simulink model "Multiuav"  (Simulink 4.00)
settings: Solver=FixedStepDiscrete  StartTime=0.0  StopTime=g_StopTime  FixedStep=g_SampleTime  RelTol=1e-3
undefined symbols (not defined in the file): ATRFunctions, g_AssignmentAlgorithm, g_CommandTurnRadius, g_CoordinationDelayDen, g_DefaultWaypointAltitude, g_EnableTarget, g_EnableVehicle, g_EntityTypes, g_MaxNumberTargets, g_MaxNumberVehicles, g_MaxReassignmentDeltaTime, g_ObjectMessageIDs, g_OptionSaveDataAVDS, g_OptionSaveDataPlot, g_SampleTime, g_SensorRollLimitDeg, g_TargetStates, g_Tasks, g_TypeAssignment, g_VehicleInputFiles, g_VehicleMemory, g_VehicleTypes, g_WaypointDefinitions, g_WaypointTypes
libraries: cooperative x42
(part 2 of 4)

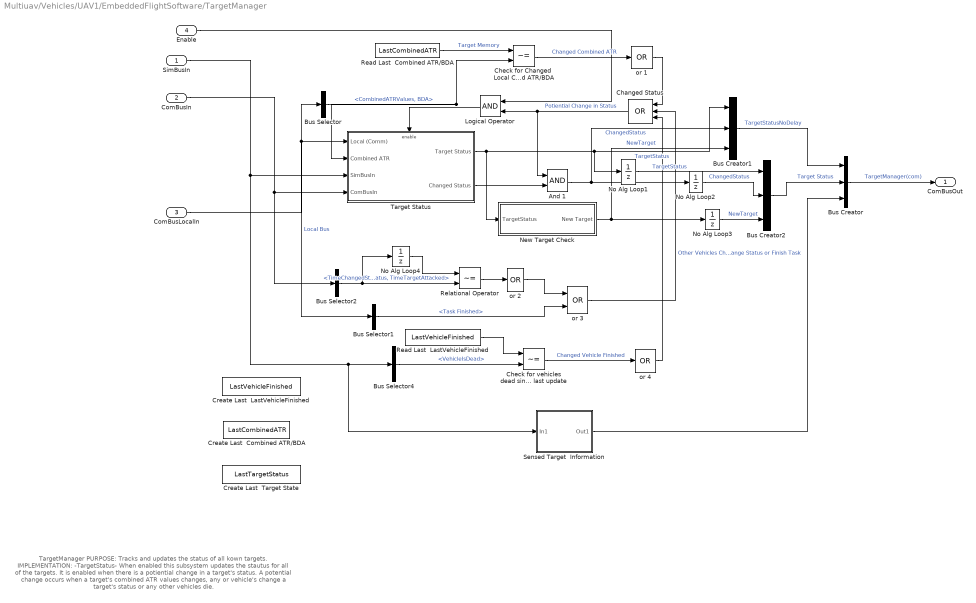
== system Multiuav/Vehicles/UAV1/EmbeddedFlightSoftware/TargetManager ==
  note: TargetManager
      |
      | PURPOSE: Tracks and updates the status of all
      |      kown targets.
      |
      | IMPLEMENTATION:
      | -TargetStatus- When enabled this subsystem updates the stautus for all of the targets.
      |      It is enabled when there is a potiential change in a target's status. A potential
      |      change occurs when a target's combined ATR values changes, any or vehicle's
      |      change a target's status or any other vehicles die.
  SimBusIn : Inport  Port=1  LatchInput=off  SampleTime=g_SampleTime
  ComBusIn : Inport  Port=2  LatchInput=off  SampleTime=g_SampleTime
  ComBusLocalIn : Inport  Port=3  LatchInput=off  SampleTime=g_SampleTime
  Enable : Inport  Port=4  LatchInput=off  SampleTime=g_SampleTime
  And 1 : Logic  Operator=AND  Inputs=2
  Bus Creator : BusCreator  Inputs=3
  Bus Creator1 : BusCreator  Inputs=3
  Bus Creator2 : BusCreator  Inputs=3
  Bus Selector : BusSelector  OutputSignals=EFS(com).SensorManager(com).ATR Combined.CombinedATRValues,EFS(com).SensorManager(com).BDA  MuxedOutput=on
  Bus Selector1 : BusSelector  OutputSignals=EFS(com).RouteManager(com).TaskStatus.Task Finished  MuxedOutput=off
  Bus Selector2 : BusSelector  OutputSignals=TimeChangedStatus,TimeTargetAttacked  MuxedOutput=on
  Bus Selector4 : BusSelector  OutputSignals=ExternalTruth.VehicleIsDead  MuxedOutput=on
  Changed Status : Logic  Orientation=left  Operator=OR  Inputs=3
  Check for Changed  Local Combined ATR/BDA : RelationalOperator  Operator=~=
  Check for vehicles dead since last update : RelationalOperator  Operator=~=
  Create Last  Combined ATR/BDA : DataStoreMemory  DataStoreName=LastCombinedATR  InitialValue=[1:(g_MaxNumberTargets*2)]*0
  Create Last  LastVehicleFinished : DataStoreMemory  DataStoreName=LastVehicleFinished  InitialValue=[1:(g_MaxNumberVehicles)]*0
  Create Last  Target State : DataStoreMemory  DataStoreName=LastTargetStatus  InitialValue=[1:(g_MaxNumberTargets)]*0
  Logical Operator : Logic  Orientation=left  Operator=AND  Inputs=2
  New Target Check : Subsystem
      settings: RTWFcnNameOpts=Auto  RTWFileNameOpts=Auto
  No Alg Loop{1..4} (4 alike) : UnitDelay  X0=0  SampleTime=g_SampleTime
      settings: RTWStateStorageClass=Auto
  Read Last  Combined ATR/BDA : DataStoreRead  DataStoreName=LastCombinedATR  SampleTime=g_SampleTime
  Read Last  LastVehicleFinished : DataStoreRead  DataStoreName=LastVehicleFinished  SampleTime=g_SampleTime
  Relational Operator : RelationalOperator  Operator=~=
  Sensed Target  Information : Subsystem
      settings: RTWFcnNameOpts=Auto  RTWFileNameOpts=Auto
  Target Status : Subsystem  TreatAsAtomicUnit=on
      settings: RTWFcnNameOpts=Auto  RTWFileNameOpts=Auto
  or 1 : Logic  Operator=OR  Inputs=1
  or 2 : Logic  Operator=OR  Inputs=1
  or 3 : Logic  Operator=OR  Inputs=2
  or 4 : Logic  Operator=OR  Inputs=1
  ComBusOut : Outport  Port=1
  wires:
  or 2/1 -> or 3/1
  No Alg Loop4/1 -> Relational Operator/1
  No Alg Loop3/1 -> Bus Creator2/3  "NewTarget"
  No Alg Loop2/1 -> Bus Creator2/2  "ChangedStatus"
  No Alg Loop1/1 -> Bus Creator2/1  "TargetStatus"
  New Target Check/1(New Target) -> No Alg Loop3/1, Bus Creator1/3  "NewTarget"
  Sensed Target  Information/1(Out1) -> Bus Creator/3
  Enable/1 -> Logical Operator/1
  Logical Operator/1 -> Target Status/Enable
  Bus Selector4/1 -> Check for vehicles dead since last update/2  "<VehicleIsDead>"
  Read Last  LastVehicleFinished/1 -> Check for vehicles dead since last update/1
  Check for vehicles dead since last update/1 -> or 4/1  "Changed Vehicle Finished"
  or 4/1 -> Changed Status/3
  or 3/1 -> Changed Status/2  "Other Vehicles Change Status or Finish Task"
  Relational Operator/1 -> or 2/1
  Bus Selector1/1 -> or 3/2  "<Task Finished>"
  Check for Changed  Local Combined ATR/BDA/1 -> or 1/1  "Changed Combined ATR"
  Target Status/1(Target Status) -> No Alg Loop1/1, Bus Creator1/1, New Target Check/1(TargetStatus)  "TargetStatus"
  Bus Creator2/1 -> Bus Creator/2  "Target Status"
  Changed Status/1 -> Logical Operator/2, And 1/1  "Potiential Change in Status"
  Bus Selector2/1 -> Relational Operator/2, No Alg Loop4/1  "<TimeChangedStatus, TimeTargetAttacked>"
  or 1/1 -> Changed Status/1
  Bus Selector/1 -> Target Status/2(Combined ATR), Check for Changed  Local Combined ATR/BDA/2  "<CombinedATRValues, BDA>"
  Read Last  Combined ATR/BDA/1 -> Check for Changed  Local Combined ATR/BDA/1  "Target Memory"
  Target Status/2(Changed Status) -> And 1/2
  And 1/1 -> Bus Creator1/2, No Alg Loop2/1  "ChangedStatus"
  ComBusIn/1 -> Bus Selector2/1, Target Status/4(ComBusIn)
  Bus Creator/1 -> ComBusOut/1  "TargetManager(com)"
  SimBusIn/1 -> Sensed Target  Information/1(In1), Bus Selector4/1, Target Status/3(SimBusIn)
  ComBusLocalIn/1 -> Bus Selector1/1, Bus Selector/1, Target Status/1(Local (Comm))  "Local Bus"
  Bus Creator1/1 -> Bus Creator/1  "TargetStatusNoDelay"

== system Multiuav/Vehicles/UAV1/EmbeddedFlightSoftware/WeaponsManager ==
  note: Weapons Manager
      |
      | PURPOSE: Selects a weapon and then simulates its deployment.
      |
      | IMPLEMENTATION:
      | -TargetBombed- calls the function "WeaponsRelease.m" which returns
      |      a unique BombID number, the type of bomb dropped and the
      |      bomb's impact coordinates.
  ComBusLocalIn : Inport  Port=1  LatchInput=off  SampleTime=g_SampleTime
  Enable : EnablePort
  Bus Creator : BusCreator  Inputs=1
  Bus Creator1 : BusCreator  Inputs=1
  Bus Creator2 : BusCreator  Inputs=4
  Bus Selector : BusSelector  OutputSignals=VehicleID,EFS(com).RouteManager(com).TaskStatus.Target Attacked,Dynamics(com).AC Dynamics.Position_x,Dynamics(com).AC Dynamics.Position_y  MuxedOutput=on
  Constant : Constant  Value=0
  Demux : Demux  Outputs=4  BusSelectionMode=off
  TargetBombed : S-Function  FunctionName=WeaponsReleaseS  Parameters='Bomb'  PortCounts=[]  SFunctionModules=''
  SimBusOut : Outport  Port=1
  ComBusOut : Outport  Port=2  InitialOutput=[0]
  wires:
  Bus Selector/1 -> TargetBombed/1  "<VehicleID, Target Attacked, Position_x, Position_y>"
  Bus Creator2/1 -> Bus Creator1/1  "BombDrop"
  Bus Creator1/1 -> SimBusOut/1  "WeaponsManager(sim)"
  Demux/4 -> Bus Creator2/4  "BombPositionY"
  Demux/3 -> Bus Creator2/3  "BombPositionX"
  Demux/2 -> Bus Creator2/2  "BombType"
  Demux/1 -> Bus Creator2/1  "BombID"
  TargetBombed/1 -> Demux/1
  Constant/1 -> Bus Creator/1  "WeaponsManagerTemp"
  Bus Creator/1 -> ComBusOut/1  "WeaponsManager(com)"
  ComBusLocalIn/1 -> Bus Selector/1

== system Multiuav/Vehicles/UAV1/ReceiveTruth/ImplementNewAssignment ==
  VehicleID : Inport  Port=1  LatchInput=off
  TruthBus : Inport  Port=2  LatchInput=off
  Constant : Constant  Value=0
  Relational Operator : RelationalOperator  Operator=<
  VehicleAlive : Subsystem  TreatAsAtomicUnit=on
      settings: RTWFcnNameOpts=Auto  RTWFileNameOpts=Auto
  wires:
  TruthBus/1 -> VehicleAlive/2(In2)
  Constant/1 -> Relational Operator/1
  VehicleID/1 -> VehicleAlive/1(In1), Relational Operator/2
  Relational Operator/1 -> VehicleAlive/Enable

== system Multiuav/Vehicles/UAV1/SaveAVDSData/SaveVehicleData for AVDS ==
  note: SaveVehicleData for AVDS
      |
      | PURPOSE: Saves vehicle state information to a text file that is suitable
      |      for playback in AVDS.
      | IMPLEMENTATION:
      | - AVDSData2WorkSpace - calls the M-function "AVDSData2WorkSpace"
      |      to save the data.
  Time : Inport  Port=1  LatchInput=off  SampleTime=g_SampleTime
  ID : Inport  Port=2  LatchInput=off  SampleTime=g_SampleTime
  Data : Inport  Port=3  LatchInput=off  SampleTime=g_SampleTime
  Vehicle Type : Inport  Port=4  LatchInput=off  SampleTime=g_SampleTime
  Enable : EnablePort
  AVDSData2WorkSpaceS : S-Function  FunctionName=AVDSData2WorkSpaceS  PortCounts=[]  SFunctionModules=''
  Mux1 : Mux  Inputs=4
  wires:
  Vehicle Type/1 -> Mux1/4
  Data/1 -> Mux1/3
  ID/1 -> Mux1/1
  Time/1 -> Mux1/2
  Mux1/1 -> AVDSData2WorkSpaceS/1

== system Multiuav/Vehicles/UAV1/SendMessages/SendATRSingle ==
  VehicleID : Inport  Port=1  LatchInput=off
  CommBusLocal : Inport  Port=2  LatchInput=off
  Bus Selector4 : BusSelector  OutputSignals=EFS(com).SensorManager(com).ATR Single.ATR Time,EFS(com).SensorManager(com).ATR Single  MuxedOutput=on
  Mux3 : Mux  Inputs=3
  SendATRSingle : cooperative/SendMessage  ReuseMatrix=growing  MessageTypeStr=ATRSingle
  Terminator : Terminator
  VehicleOffset : Constant  Value=g_ObjectMessageIDs.AllVehiclesTypeShifted + 1
  wires:
  CommBusLocal/1 -> Bus Selector4/1
  VehicleID/1 -> Mux3/1
  Mux3/1 -> SendATRSingle/1
  Bus Selector4/1 -> Mux3/2  "<ATR Time, ATR Single>"
  VehicleOffset/1 -> Mux3/3
  SendATRSingle/1 -> Terminator/1

== system Multiuav/Vehicles/UAV1/SendMessages/SendATRTime ==
  VehicleID : Inport  Port=1  LatchInput=off
  CommBusLocal : Inport  Port=2  LatchInput=off
  Bus Selector1 : BusSelector  OutputSignals=EFS(com).SensorManager(com).ATR Single.ATR Time  MuxedOutput=off
  CreateWaypointIndex : DataStoreMemory  DataStoreName=ATRTime  InitialValue=0
  Enabled Subsystem : Subsystem  TreatAsAtomicUnit=on
      settings: RTWFcnNameOpts=Auto  RTWFileNameOpts=Auto
  Mux2 : Mux  Inputs=4
  ReadWaypointIndex : DataStoreRead  DataStoreName=ATRTime  SampleTime=g_SampleTime
  Relational Operator : RelationalOperator  Operator=~=
  SendATRTime : cooperative/SendMessage  ReuseMatrix=growing  MessageTypeStr=ATRTime
  Terminator : Terminator
  VehicleOffset : Constant  Value=g_ObjectMessageIDs.AllVehiclesTypeShifted + 1
  wires:
  Bus Selector1/1 -> Enabled Subsystem/1(ATRTime), Relational Operator/2, Mux2/3  "<ATR Time>"
  Enabled Subsystem/1(TimeStamp) -> Mux2/2  "TimeStamp"
  Mux2/1 -> SendATRTime/1
  Relational Operator/1 -> Enabled Subsystem/Enable
  ReadWaypointIndex/1 -> Relational Operator/1
  VehicleID/1 -> Mux2/1
  CommBusLocal/1 -> Bus Selector1/1
  VehicleOffset/1 -> Mux2/4
  SendATRTime/1 -> Terminator/1

== system Multiuav/Vehicles/UAV1/SendMessages/SendAuctionData ==
  VehicleID : Inport  Port=1  LatchInput=off
  CommBusLocal : Inport  Port=2  LatchInput=off
  Bus Selector1 : BusSelector  OutputSignals=EFS(com).CooperationManager(com).AuctionData.MessageNumber,EFS(com).CooperationManager(com).AuctionData.ReplanRound,EFS(com).CooperationManager(com).AuctionData.BidTarget,EFS(com).CooperationManager(com).AuctionData.BidPrice,EFS(com).CooperationManager(com).AuctionData.BidTargetETA,EFS(com).CooperationManager(com).AuctionData.AssignedTarget,EFS(com).CooperationManager(com).AuctionData.AssignedPrice,EFS(com).CooperationManager(com).AuctionData.AssignedTargetETA  MuxedOutput=off
  Data Store Memory : DataStoreMemory  DataStoreName=LastMessageNumber  InitialValue=0
  Data Store Read : DataStoreRead  DataStoreName=LastMessageNumber  SampleTime=g_SampleTime
  Enabled Subsystem : Subsystem  Priority=1  TreatAsAtomicUnit=on
      settings: RTWFcnNameOpts=Auto  RTWFileNameOpts=Auto
  Mux2 : Mux  Inputs=11
  Relational Operator : RelationalOperator  Operator=~=
  "SendAuctionData " : cooperative/SendMessage  Priority=2  ReuseMatrix=growing  MessageTypeStr=AuctionData
  Sum : Sum  Inputs=+  SaturateOnIntegerOverflow=on
  Terminator : Terminator
  VehicleOffset : Constant  Value=g_ObjectMessageIDs.AllVehiclesTypeShifted + 1
  wires:
  Bus Selector1/1 -> Enabled Subsystem/1(MessageNumber), Relational Operator/2  "<MessageNumber>"
  Bus Selector1/2 -> Mux2/4  "<ReplanRound>"
  Bus Selector1/3 -> Mux2/5  "<BidTarget>"
  Bus Selector1/4 -> Mux2/6  "<BidPrice>"
  Bus Selector1/5 -> Mux2/7  "<BidTargetETA>"
  Bus Selector1/6 -> Mux2/8  "<AssignedTarget>"
  Bus Selector1/7 -> Mux2/9  "<AssignedPrice>"
  Bus Selector1/8 -> Mux2/10  "<AssignedTargetETA>"
  Sum/1 -> Enabled Subsystem/Enable
  Relational Operator/1 -> Sum/1
  Data Store Read/1 -> Relational Operator/1
  Enabled Subsystem/1(TimeStamp) -> Mux2/3, Mux2/2  "TimeStamp"
  Mux2/1 -> "SendAuctionData "/1
  VehicleID/1 -> Mux2/1
  CommBusLocal/1 -> Bus Selector1/1
  VehicleOffset/1 -> Mux2/11
  "SendAuctionData "/1 -> Terminator/1

== system Multiuav/Vehicles/UAV1/SendMessages/SendChangedStatus ==
  VehicleID : Inport  Port=1  LatchInput=off
  CommBusLocal : Inport  Port=2  LatchInput=off
  Bus Selector1 : BusSelector  OutputSignals=EFS(com).TargetManager(com).Target Status.ChangedStatus  MuxedOutput=off
  Enabled Subsystem : Subsystem  TreatAsAtomicUnit=on
      settings: RTWFcnNameOpts=Auto  RTWFileNameOpts=Auto
  Mux2 : Mux  Inputs=4
  "SendChangedStatus " : cooperative/SendMessage  ReuseMatrix=growing  MessageTypeStr=ChangedStatus
  Terminator : Terminator
  VehicleOffset : Constant  Value=g_ObjectMessageIDs.AllVehiclesTypeShifted + 1
  wires:
  Bus Selector1/1 -> Enabled Subsystem/Enable, Mux2/3  "<ChangedStatus>"
  Enabled Subsystem/1(TimeStamp) -> Mux2/2  "TimeStamp"
  Mux2/1 -> "SendChangedStatus "/1
  VehicleID/1 -> Mux2/1
  CommBusLocal/1 -> Bus Selector1/1
  VehicleOffset/1 -> Mux2/4
  "SendChangedStatus "/1 -> Terminator/1

== system Multiuav/Vehicles/UAV1/SendMessages/SendETAsCostsReturnToSearch ==
  VehicleID : Inport  Port=1  LatchInput=off
  CommBusLocal : Inport  Port=2  LatchInput=off
  Bus Selector2 : BusSelector  OutputSignals=EFS(com).RouteManager(com).Replan ETAs and Costs.ReplanTime,EFS(com).RouteManager(com).Replan ETAs and Costs  MuxedOutput=on
  Mux : Mux  Inputs=3
  SendETAsCostsReturnToSearch : cooperative/SendMessage  ReuseMatrix=growing  MessageTypeStr=ETACostToSearch
  Terminator : Terminator
  VehicleOffset : Constant  Value=g_ObjectMessageIDs.AllVehiclesTypeShifted + 1
  wires:
  CommBusLocal/1 -> Bus Selector2/1
  VehicleID/1 -> Mux/1
  Mux/1 -> SendETAsCostsReturnToSearch/1
  Bus Selector2/1 -> Mux/2  "<ReplanTime, Replan ETAs and Costs>"
  VehicleOffset/1 -> Mux/3
  SendETAsCostsReturnToSearch/1 -> Terminator/1

== system Multiuav/Vehicles/UAV1/SendMessages/SendPositionFlag ==
  VehicleID : Inport  Port=1  LatchInput=off
  CommBusLocal : Inport  Port=2  LatchInput=off
  CommBus : Inport  Port=3  LatchInput=off
  Bus Selector1 : BusSelector  OutputSignals=EFS(com).TargetManager(com).Target Status.NewTarget,EFS(com).RouteManager(com).NewPlans  MuxedOutput=on
  Bus Selector2 : BusSelector  OutputSignals=TimeTriggerReplan  MuxedOutput=on
  CreateWaypointIndex : DataStoreMemory  DataStoreName=PositionFlag  InitialValue=[0 0 0]
  Enabled Subsystem : Subsystem  TreatAsAtomicUnit=on
      settings: RTWFcnNameOpts=Auto  RTWFileNameOpts=Auto
  Logical Operator1 : Logic  Operator=OR  Inputs=1
  Mux : Mux  Inputs=2
  Mux2 : Mux  Inputs=4
  ReadWaypointIndex : DataStoreRead  DataStoreName=PositionFlag  SampleTime=g_SampleTime
  Relational Operator : RelationalOperator  Operator=~=
  SendATRTime : cooperative/SendMessage  ReuseMatrix=growing  MessageTypeStr=SendPositionsFlag
  Terminator : Terminator
  VehicleOffset : Constant  Value=g_ObjectMessageIDs.AllVehiclesTypeShifted + 1
  wires:
  Mux/1 -> Enabled Subsystem/1(PositionFlag), Relational Operator/2
  Bus Selector1/1 -> Mux/1  "<NewTarget, NewPlans>"
  Bus Selector2/1 -> Mux/2  "<TimeTriggerReplan>"
  CommBus/1 -> Bus Selector2/1
  Logical Operator1/1 -> Mux2/3, Enabled Subsystem/Enable
  Relational Operator/1 -> Logical Operator1/1
  CommBusLocal/1 -> Bus Selector1/1
  VehicleID/1 -> Mux2/1
  ReadWaypointIndex/1 -> Relational Operator/1
  Mux2/1 -> SendATRTime/1
  Enabled Subsystem/1(TimeStamp) -> Mux2/2  "TimeStamp"
  VehicleOffset/1 -> Mux2/4
  SendATRTime/1 -> Terminator/1

== system Multiuav/Vehicles/UAV1/SendMessages/SendPositionID ==
  note: NOTE: Since the received messages are not reset to zero after they are handled, it was necessary to reset the PositionsFlag signal here.
      | The issue of resetting the message values to zero may be moved into the S-Function.
  VehicleID : Inport  Port=1  LatchInput=off
  CommBusLocal : Inport  Port=2  LatchInput=off
  CommBus : Inport  Port=3  LatchInput=off
  Bus Selector1 : BusSelector  OutputSignals=Dynamics(com).AC Dynamics.Position_x,Dynamics(com).AC Dynamics.Position_y,Dynamics(com).AC Dynamics.Psi  MuxedOutput=on
  Bus Selector2 : BusSelector  OutputSignals=TimePositionsFlag  MuxedOutput=on
  Data Store Memory : DataStoreMemory  DataStoreName=PositionsSendFlagTime  InitialValue=0
  Data Store Read : DataStoreRead  DataStoreName=PositionsSendFlagTime  SampleTime=g_SampleTime
  Enabled Subsystem : Subsystem  TreatAsAtomicUnit=on
      settings: RTWFcnNameOpts=Auto  RTWFileNameOpts=Auto
  Mux2 : Mux  Inputs=5
  Relational Operator : RelationalOperator  Operator=~=
  "SendPositionID " : cooperative/SendMessage  ReuseMatrix=growing  MessageTypeStr=PositionID
  Terminator : Terminator
  VehicleOffset : Constant  Value=g_ObjectMessageIDs.AllVehiclesTypeShifted + 1
  wires:
  Relational Operator/1 -> Enabled Subsystem/Enable
  Data Store Read/1 -> Relational Operator/1
  Bus Selector2/1 -> Relational Operator/2, Enabled Subsystem/1(PositionSendFlag Time)  "<TimePositionsFlag>"
  CommBus/1 -> Bus Selector2/1
  CommBusLocal/1 -> Bus Selector1/1
  VehicleID/1 -> Mux2/3, Mux2/1
  Mux2/1 -> "SendPositionID "/1
  Enabled Subsystem/1(TimeStamp) -> Mux2/2  "TimeStamp"
  Bus Selector1/1 -> Mux2/4  "<Position_x, Position_y, Psi>"
  VehicleOffset/1 -> Mux2/5
  "SendPositionID "/1 -> Terminator/1

== system Multiuav/Vehicles/UAV1/SendMessages/SendTargetAttacked ==
  VehicleID : Inport  Port=1  LatchInput=off
  CommBusLocal : Inport  Port=2  LatchInput=off
  Bus Selector1 : BusSelector  OutputSignals=EFS(com).RouteManager(com).TaskStatus.Target Attacked  MuxedOutput=off
  CreateWaypointIndex : DataStoreMemory  DataStoreName=TargetAttacked  InitialValue=0
  Enabled Subsystem : Subsystem  TreatAsAtomicUnit=on
      settings: RTWFcnNameOpts=Auto  RTWFileNameOpts=Auto
  Mux2 : Mux  Inputs=4
  ReadWaypointIndex : DataStoreRead  DataStoreName=TargetAttacked  SampleTime=g_SampleTime
  Relational Operator : RelationalOperator  Operator=~=
  "SendTargetAttacked " : cooperative/SendMessage  ReuseMatrix=growing  MessageTypeStr=TargetAttacked
  Terminator : Terminator
  VehicleOffset : Constant  Value=g_ObjectMessageIDs.AllVehiclesTypeShifted + 1
  wires:
  CommBusLocal/1 -> Bus Selector1/1
  VehicleID/1 -> Mux2/1
  ReadWaypointIndex/1 -> Relational Operator/1
  Relational Operator/1 -> Enabled Subsystem/Enable
  Mux2/1 -> "SendTargetAttacked "/1
  Enabled Subsystem/1(TimeStamp) -> Mux2/2  "TimeStamp"
  Bus Selector1/1 -> Mux2/3, Relational Operator/2, Enabled Subsystem/1("TargetAttacked ")  "<Target Attacked>"
  VehicleOffset/1 -> Mux2/4
  "SendTargetAttacked "/1 -> Terminator/1

== system Multiuav/Vehicles/UAV1/SendMessages/SendTargetStatus ==
  VehicleID : Inport  Port=1  LatchInput=off
  CommBusLocal : Inport  Port=2  LatchInput=off
  Bus Selector1 : BusSelector  OutputSignals=EFS(com).TargetManager(com).TargetStatusNoDelay.TargetStatus  MuxedOutput=off
  Bus Selector2 : BusSelector  OutputSignals=EFS(com).TargetManager(com).TargetStatusNoDelay.ChangedStatus  MuxedOutput=off
  Enabled Subsystem : Subsystem  Priority=1  TreatAsAtomicUnit=on
      settings: RTWFcnNameOpts=Auto  RTWFileNameOpts=Auto
  Mux2 : Mux  Inputs=4
  "SendTargetStatus " : cooperative/SendMessage  Priority=2  ReuseMatrix=growing  MessageTypeStr=TargetStatus
  Terminator : Terminator
  VehicleOffset : Constant  Value=g_ObjectMessageIDs.AllVehiclesTypeShifted + 1
  wires:
  Bus Selector2/1 -> Enabled Subsystem/Enable  "<ChangedStatus>"
  Bus Selector1/1 -> Mux2/3  "<TargetStatus>"
  Enabled Subsystem/1(TimeStamp) -> Mux2/2  "TimeStamp"
  Mux2/1 -> "SendTargetStatus "/1
  VehicleID/1 -> Mux2/1
  CommBusLocal/1 -> Bus Selector2/1, Bus Selector1/1
  VehicleOffset/1 -> Mux2/4
  "SendTargetStatus "/1 -> Terminator/1

== system Multiuav/Vehicles/UAV1/SendMessages/SendTaskBenefits ==
  VehicleID : Inport  Port=1  LatchInput=off
  CommBusLocal : Inport  Port=2  LatchInput=off
  Bus Selector1 : BusSelector  OutputSignals=EFS(com).CooperationManager(com).Algorithm Data.ReplanRound,EFS(com).CooperationManager(com).Algorithm Data.TargetStates,EFS(com).CooperationManager(com).Algorithm Data.TaskBenefits,EFS(com).CooperationManager(com).Algorithm Data.TimeToComplete,EFS(com).CooperationManager(com).Algorithm Data.SearchBenefit  MuxedOutput=off
  Data Store Memory : DataStoreMemory  DataStoreName=LastReplanRound  InitialValue=[0;0]
  Data Store Read : DataStoreRead  DataStoreName=LastReplanRound  SampleTime=g_SampleTime
  Enabled Subsystem : Subsystem  Priority=1  TreatAsAtomicUnit=on
      settings: RTWFcnNameOpts=Auto  RTWFileNameOpts=Auto
  Mux2 : Mux  Inputs=8
  Relational Operator : RelationalOperator  Operator=~=
  "SendTaskBenefits " : cooperative/SendMessage  Priority=2  ReuseMatrix=growing  MessageTypeStr=TaskBenefits
  Sum : Sum  Inputs=+  SaturateOnIntegerOverflow=on
  Terminator : Terminator
  VehicleOffset : Constant  Value=g_ObjectMessageIDs.AllVehiclesTypeShifted + 1
  wires:
  Bus Selector1/5 -> Mux2/7  "<SearchBenefit>"
  Bus Selector1/4 -> Mux2/6  "<TimeToComplete>"
  Bus Selector1/3 -> Mux2/5  "<TaskBenefits>"
  Sum/1 -> Enabled Subsystem/Enable
  Relational Operator/1 -> Sum/1
  Data Store Read/1 -> Relational Operator/1
  Bus Selector1/2 -> Mux2/4  "<TargetStates>"
  Bus Selector1/1 -> Enabled Subsystem/1(ReplanRound), Relational Operator/2, Mux2/3  "<ReplanRound>"
  Enabled Subsystem/1(TimeStamp) -> Mux2/2  "TimeStamp"
  Mux2/1 -> "SendTaskBenefits "/1
  VehicleID/1 -> Mux2/1
  CommBusLocal/1 -> Bus Selector1/1
  VehicleOffset/1 -> Mux2/8
  "SendTaskBenefits "/1 -> Terminator/1

== system Multiuav/Vehicles/UAV1/SendMessages/SendTriggerReplan ==
  VehicleID : Inport  Port=1  LatchInput=off
  CommBusLocal : Inport  Port=2  LatchInput=off
  Bus Selector1 : BusSelector  OutputSignals=EFS(com).RouteManager(com).TaskStatus.TriggerReplan  MuxedOutput=on
  Enabled Subsystem : Subsystem  TreatAsAtomicUnit=on
      settings: RTWFcnNameOpts=Auto  RTWFileNameOpts=Auto
  Mux1 : Mux  Inputs=4
  SendTriggerReplan : cooperative/SendMessage  ReuseMatrix=growing  MessageTypeStr=TriggerReplan
  Terminator : Terminator
  VehicleOffset : Constant  Value=g_ObjectMessageIDs.AllVehiclesTypeShifted + 1
  wires:
  Enabled Subsystem/1(TimeStamp) -> Mux1/2  "TriggerReplanTriggered"
  Bus Selector1/1 -> Enabled Subsystem/Enable, Mux1/3  "<TriggerReplan>"
  CommBusLocal/1 -> Bus Selector1/1
  VehicleID/1 -> Mux1/1
  Mux1/1 -> SendTriggerReplan/1
  VehicleOffset/1 -> Mux1/4
  SendTriggerReplan/1 -> Terminator/1

== system Multiuav/Vehicles/UAV1/SendMessages/SendWaypointNumber ==
  VehicleID : Inport  Port=1  LatchInput=off
  CommBusLocal : Inport  Port=2  LatchInput=off
  Bus Selector1 : BusSelector  OutputSignals=Dynamics(com).TacticalManuevering.WayPointNumber  MuxedOutput=off
  CreateWaypointIndex : DataStoreMemory  DataStoreName=WaypoinNumber  InitialValue=1
  Enabled Subsystem : Subsystem  TreatAsAtomicUnit=on
      settings: RTWFcnNameOpts=Auto  RTWFileNameOpts=Auto
  Mux2 : Mux  Inputs=4
  ReadWaypointIndex : DataStoreRead  DataStoreName=WaypoinNumber  SampleTime=g_SampleTime
  Relational Operator : RelationalOperator  Operator=~=
  SendWaypointIndex : cooperative/SendMessage  ReuseMatrix=growing  MessageTypeStr=WaypointIndex
  Terminator : Terminator
  VehicleOffset : Constant  Value=g_ObjectMessageIDs.AllVehiclesTypeShifted + 1
  wires:
  CommBusLocal/1 -> Bus Selector1/1
  VehicleID/1 -> Mux2/1
  ReadWaypointIndex/1 -> Relational Operator/1
  Relational Operator/1 -> Enabled Subsystem/Enable
  Mux2/1 -> SendWaypointIndex/1
  Enabled Subsystem/1(TimeStamp) -> Mux2/2  "TimeStamp"
  Bus Selector1/1 -> Mux2/3, Relational Operator/2, Enabled Subsystem/1(Waypoint)  "<WayPointNumber>"
  VehicleOffset/1 -> Mux2/4
  SendWaypointIndex/1 -> Terminator/1

== system Multiuav/Vehicles/UAV1/SendTruth/SendNewAssignment ==
  VehicleID : Inport  Port=1  LatchInput=off
  SimmBusLocal : Inport  Port=2  LatchInput=off
  Bus Selector1 : BusSelector  OutputSignals=EFS(sim).CooperationManager(com).NewAssignmentTime  MuxedOutput=off
  Changed1 : Subsystem
      settings: RTWFcnNameOpts=Auto  RTWFileNameOpts=Auto
  Enabled Subsystem : Subsystem  TreatAsAtomicUnit=on
      settings: RTWFcnNameOpts=Auto  RTWFileNameOpts=Auto
  Mux2 : Mux  Inputs=4
  Recipients : Constant  Value=[g_ObjectMessageIDs.AllVehiclesTypeShifted + 1]
  "SendTruth " : cooperative/SendTruth   ReuseMatrix=growing  MessageTypeStr=ChangeAssignmentFlagSelf
  Terminator : Terminator
  wires:
  "SendTruth "/1 -> Terminator/1
  Bus Selector1/1 -> Mux2/3, Changed1/1(Signal)  "<NewAssignmentTime>"
  Enabled Subsystem/1(TimeStamp) -> Mux2/2  "TimeStamp"
  Mux2/1 -> "SendTruth "/1
  VehicleID/1 -> Mux2/1
  Recipients/1 -> Mux2/4
  SimmBusLocal/1 -> Bus Selector1/1
  Changed1/1(Greater?) -> Enabled Subsystem/Enable

== system Multiuav/Vehicles/UAV1/SendTruth/SendTargetStatus ==
  VehicleID : Inport  Port=1  LatchInput=off
  CommBusLocal : Inport  Port=2  LatchInput=off
  Bus Selector2 : BusSelector  OutputSignals=EFS(com).TargetManager(com).Target Status.TargetStatus  MuxedOutput=off
  Data Store Memory : DataStoreMemory  DataStoreName=TargetStatus  InitialValue=zeros(g_MaxNumberTargets,1)
  Data Store Read : DataStoreRead  DataStoreName=TargetStatus  SampleTime=g_SampleTime
  Enabled Subsystem : Subsystem  TreatAsAtomicUnit=on
      settings: RTWFcnNameOpts=Auto  RTWFileNameOpts=Auto
  Mux2 : Mux  Inputs=4
  Recipients : Constant  Value=g_ObjectMessageIDs.DataSaveID + g_ObjectMessageIDs.MiscTypeShifted
  Relational Operator : RelationalOperator  Operator=~=
  "SendTruth " : cooperative/SendTruth   ReuseMatrix=static  MessageTypeStr=TargetStatus
  Terminator : Terminator
  wires:
  Data Store Read/1 -> Relational Operator/1
  Relational Operator/1 -> Enabled Subsystem/Enable
  Enabled Subsystem/1(TimeStamp) -> Mux2/2  "TimeStamp"
  Mux2/1 -> "SendTruth "/1
  VehicleID/1 -> Mux2/1
  Recipients/1 -> Mux2/4
  CommBusLocal/1 -> Bus Selector2/1
  Bus Selector2/1 -> Mux2/3, Relational Operator/2, Enabled Subsystem/1(TargetStatus)  "<TargetStatus>"
  "SendTruth "/1 -> Terminator/1

== system Multiuav/Vehicles/UAV1/SendTruth/SendTrackList ==
  VehicleID : Inport  Port=1  LatchInput=off
  CommBusLocal : Inport  Port=2  LatchInput=off
  Bus Selector1 : BusSelector  OutputSignals=Dynamics(com).SensedTargets.SensedTargets,EFS(com).TargetManager(com).SensedTargetInformation.Targets  MuxedOutput=on
  Data Store Memory : DataStoreMemory  DataStoreName=TrackList  InitialValue=zeros(7*g_MaxNumberTargets,1)
  Data Store Read : DataStoreRead  DataStoreName=TrackList  SampleTime=g_SampleTime
  Enabled Subsystem : Subsystem  TreatAsAtomicUnit=on
      settings: RTWFcnNameOpts=Auto  RTWFileNameOpts=Auto
  Mux : Mux  Inputs=2
  Mux2 : Mux  Inputs=5
  ObjectMode_temp : Constant  Value=1
  ObjectType_temp : Constant  Value=1
  Recipients : Constant  Value=g_ObjectMessageIDs.AllVehiclesTypeShifted + 1
  Relational Operator : RelationalOperator  Operator=~=
  "SendTruth " : cooperative/SendTruth   ReuseMatrix=static  MessageTypeStr=TrackList
  Terminator : Terminator
  wires:
  Bus Selector1/1 -> Mux2/3, Enabled Subsystem/1(TrackList), Relational Operator/2  "<SensedTargets, Targets>"
  Mux2/1 -> "SendTruth "/1
  VehicleID/1 -> Mux2/1
  CommBusLocal/1 -> Bus Selector1/1
  Recipients/1 -> Mux2/5
  Data Store Read/1 -> Relational Operator/1
  Relational Operator/1 -> Enabled Subsystem/Enable
  Enabled Subsystem/1(TimeStamp) -> Mux2/2
  "SendTruth "/1 -> Terminator/1
  Mux/1 -> Mux2/4
  ObjectMode_temp/1 -> Mux/2
  ObjectType_temp/1 -> Mux/1

== system Multiuav/Vehicles/UAV1/SendTruth/SendTrueVehicleState ==
  VehicleID : Inport  Port=1  LatchInput=off
  CommBusLocal : Inport  Port=2  LatchInput=off
  SimmBusLocal : Inport  Port=3  LatchInput=off
  Bus Selector1 : BusSelector  OutputSignals=Dynamics(com).AC Dynamics.Position_x,Dynamics(com).AC Dynamics.Position_y,Dynamics(com).AC Dynamics.Altitude,Dynamics(com).AC Dynamics.Phi,Dynamics(com).AC Dynamics.Theta,Dynamics(com).AC Dynamics.Psi  MuxedOutput=on
  Bus Selector2 : BusSelector  OutputSignals=EFS(sim).RouteManager(sim).VehicleFinished.Vehicle FinishedNoDelay  MuxedOutput=on
  Digital Clock : DigitalClock  SampleTime=g_SampleTime
  Mux2 : Mux  Inputs=5
  Recipients : Constant  Value=[g_ObjectMessageIDs.AllTargetsTypeShifted + 1,g_ObjectMessageIDs.DataSaveID + g_ObjectMessageIDs.MiscTypeShifted]
  "SendTruth " : cooperative/SendTruth   ReuseMatrix=static  MessageTypeStr=VehicleState
  Terminator : Terminator
  wires:
  Bus Selector1/1 -> Mux2/3  "<Position_x, Position_y, Altitude, Phi, Theta, Psi>"
  Digital Clock/1 -> Mux2/2  "TimeStamp"
  Mux2/1 -> "SendTruth "/1
  VehicleID/1 -> Mux2/1
  CommBusLocal/1 -> Bus Selector1/1
  Recipients/1 -> Mux2/5
  "SendTruth "/1 -> Terminator/1
  SimmBusLocal/1 -> Bus Selector2/1
  Bus Selector2/1 -> Mux2/4  "<Vehicle FinishedNoDelay>"

== system Multiuav/Vehicles/UAV1/SendTruth/SendVehicleIsDead ==
  VehicleID : Inport  Port=1  LatchInput=off
  SimmBusLocal : Inport  Port=2  LatchInput=off
  Bus Selector2 : BusSelector  OutputSignals=EFS(sim).RouteManager(sim).VehicleFinished.Vehicle FinishedNoDelay  MuxedOutput=on
  Create : DataStoreMemory  DataStoreName=VehicleIDead  InitialValue=0
  Enabled Subsystem : Subsystem  TreatAsAtomicUnit=on
      settings: RTWFcnNameOpts=Auto  RTWFileNameOpts=Auto
  Mux2 : Mux  Inputs=3
  Read : DataStoreRead  DataStoreName=VehicleIDead  SampleTime=g_SampleTime
  Relational Operator : RelationalOperator  Operator=~=
  "SendTruth " : cooperative/SendTruth   ReuseMatrix=static  MessageTypeStr=VehicleIsDead
  Terminator : Terminator
  wires:
  Bus Selector2/1 -> Mux2/3, Relational Operator/2, Enabled Subsystem/1(State)  "<Vehicle FinishedNoDelay>"
  SimmBusLocal/1 -> Bus Selector2/1
  VehicleID/1 -> Mux2/1
  Mux2/1 -> "SendTruth "/1
  Relational Operator/1 -> Enabled Subsystem/Enable
  Read/1 -> Relational Operator/1
  Enabled Subsystem/1(TimeStamp) -> Mux2/2
  "SendTruth "/1 -> Terminator/1

== system Multiuav/Vehicles/UAV1/SendTruth/SendWeaponsRelease ==
  VehicleID : Inport  Port=1  LatchInput=off
  SimmBusLocal : Inport  Port=2  LatchInput=off
  Bus Selector1 : BusSelector  OutputSignals=EFS(sim).WeaponsManager(sim).BombDrop.BombID  MuxedOutput=off
  Bus Selector2 : BusSelector  OutputSignals=EFS(sim).WeaponsManager(sim).BombDrop  MuxedOutput=off
  Data Store Memory : DataStoreMemory  DataStoreName=WeaponID  InitialValue=0
  Data Store Read : DataStoreRead  DataStoreName=WeaponID  SampleTime=g_SampleTime
  Enabled Subsystem : Subsystem  TreatAsAtomicUnit=on
      settings: RTWFcnNameOpts=Auto  RTWFileNameOpts=Auto
  Mux2 : Mux  Inputs=4
  Recipients : Constant  Value=[g_ObjectMessageIDs.AllTargetsTypeShifted + 1]
  Relational Operator : RelationalOperator  Operator=~=
  "SendTruth " : cooperative/SendTruth   ReuseMatrix=static  MessageTypeStr=WeaponsRelease
  Terminator : Terminator
  wires:
  SimmBusLocal/1 -> Bus Selector1/1, Bus Selector2/1
  Recipients/1 -> Mux2/4
  VehicleID/1 -> Mux2/1
  Mux2/1 -> "SendTruth "/1
  Enabled Subsystem/1(TimeStamp) -> Mux2/2  "TimeStamp"
  Relational Operator/1 -> Enabled Subsystem/Enable
  Data Store Read/1 -> Relational Operator/1
  Bus Selector1/1 -> Relational Operator/2, Enabled Subsystem/1(WeaponID)  "<BombID>"
  Bus Selector2/1 -> Mux2/3  "<BombDrop>"
  "SendTruth "/1 -> Terminator/1

== system Multiuav/Vehicles/UAV1/SendTruth/VehicleStateSaveData ==
  VehicleID : Inport  Port=1  LatchInput=off
  CommBusLocal : Inport  Port=2  LatchInput=off
  SimmBusLocal : Inport  Port=3  LatchInput=off
  Bus Selector1 : BusSelector  OutputSignals=Dynamics(com).AC Dynamics.Position_x,Dynamics(com).AC Dynamics.Position_y,Dynamics(com).AC Dynamics.Altitude,Dynamics(com).AC Dynamics.Phi,Dynamics(com).AC Dynamics.Theta,Dynamics(com).AC Dynamics.Psi,Dynamics(com).AC Dynamics.SensorOn,Dynamics(com).TacticalManuevering.RabbitNpos,Dynamics(com).TacticalManuevering.RabbitEpos,Dynamics(com).TacticalManuevering.RabbitHdg,Dynamics(com).TacticalManuevering.AssignedTarget  MuxedOutput=on
  Bus Selector2 : BusSelector  OutputSignals=EFS(sim).RouteManager(sim).VehicleFinished.Vehicle FinishedNoDelay  MuxedOutput=on
  Digital Clock : DigitalClock  SampleTime=g_SampleTime
  Mux2 : Mux  Inputs=5
  Recipients : Constant  Value=g_ObjectMessageIDs.DataSaveID + g_ObjectMessageIDs.MiscTypeShifted
  "SendTruth " : cooperative/SendTruth   ReuseMatrix=static  MessageTypeStr=VehicleStateSaveData
  Terminator : Terminator
  wires:
  Bus Selector2/1 -> Mux2/4  "<Vehicle FinishedNoDelay>"
  SimmBusLocal/1 -> Bus Selector2/1
  Recipients/1 -> Mux2/5
  CommBusLocal/1 -> Bus Selector1/1
  VehicleID/1 -> Mux2/1
  Mux2/1 -> "SendTruth "/1
  Digital Clock/1 -> Mux2/2  "TimeStamp"
  Bus Selector1/1 -> Mux2/3  "<Position_x, Position_y, Altitude, Phi, Theta, Psi, SensorOn, RabbitNpos, RabbitEpos, RabbitHdg, AssignedTarget>"
  "SendTruth "/1 -> Terminator/1

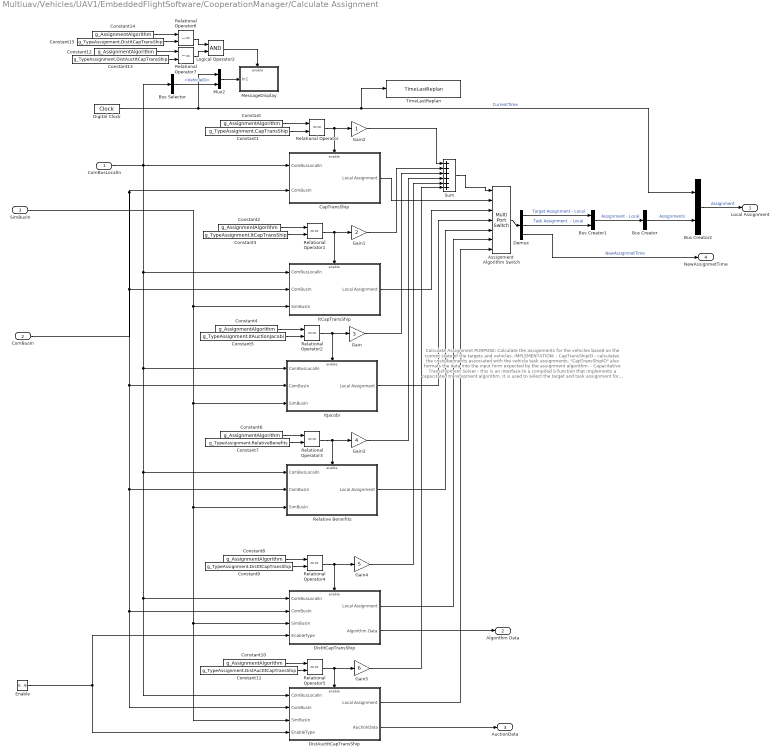
== system Multiuav/Vehicles/UAV1/EmbeddedFlightSoftware/CooperationManager/Calculate Assignment ==
  note: Calculate Assignment
      |
      | PURPOSE: Calculate the assignments for the vehicles based on the current
      |      state of the targets and vehicles.
      |
      | IMPLEMENTATION:
      | - CapTransShipIO - calculates the costs/bennefits associated with the vehicle
      |      task assignments. "CapTransShipIO" also formats the data into the input
      |      form expected by the assignment algorithm.
      | - Capacitative Transshipment Solver - this is an interface to a compiled S-function
      |      that implements a capacitated transhipment algorithm. It is used to select the
      |      target and task assignment for all of the vehicles.
      | - Assignment for Local Vehicle - uses the current vehicle's ID to select and output
      |      the target and task assignment for this vehicle.
  ComBusLocalIn : Inport  Port=1  LatchInput=off  SampleTime=g_SampleTime
  ComBusIn : Inport  Port=2  LatchInput=off  SampleTime=g_SampleTime
  SimBusIn : Inport  Port=3  LatchInput=off  SampleTime=g_SampleTime
  Enable : EnablePort  ShowOutputPort=on
  Assignment  Algorithm Switch : MultiPortSwitch  Inputs=6
  Bus Creator : BusCreator  Inputs=1
  Bus Creator1 : BusCreator  Inputs=2
  Bus Creator2 : BusCreator  Inputs=2
  Bus Selector : BusSelector  OutputSignals=VehicleID  MuxedOutput=off
  CapTransShip : Subsystem  TreatAsAtomicUnit=on
      settings: RTWFcnNameOpts=Auto  RTWFileNameOpts=Auto
  Constant{,2,4,6,8,10,12,14} (8 alike) : Constant  Value=g_AssignmentAlgorithm
  Constant1 : Constant  Value=g_TypeAssignment.CapTransShip
  Constant11 : Constant  Value=g_TypeAssignment.DistAuctItCapTransShip
  Constant13 : Constant  Value=g_TypeAssignment.DistAuctItCapTransShip
  Constant15 : Constant  Value=g_TypeAssignment.DistItCapTransShip
  Constant3 : Constant  Value=g_TypeAssignment.ItCapTransShip
  Constant5 : Constant  Value=g_TypeAssignment.ItAuctionJacobi
  Constant7 : Constant  Value=g_TypeAssignment.RelativeBenefits
  Constant9 : Constant  Value=g_TypeAssignment.DistItCapTransShip
  Demux : Demux  Outputs=3  BusSelectionMode=off
  Digital Clock : DigitalClock  SampleTime=g_SampleTime
  DistAuctItCapTransShip : Subsystem  TreatAsAtomicUnit=on
      settings: RTWFcnNameOpts=Auto  RTWFileNameOpts=Auto
  DistItCapTransShip : Subsystem  TreatAsAtomicUnit=on
      settings: RTWFcnNameOpts=Auto  RTWFileNameOpts=Auto
  Gain : Gain  Gain=3  Multiplication=Element-wise(K.*u)  SaturateOnIntegerOverflow=on
  Gain1 : Gain  Gain=2  Multiplication=Element-wise(K.*u)  SaturateOnIntegerOverflow=on
  Gain2 : Gain  Gain=1  Multiplication=Element-wise(K.*u)  SaturateOnIntegerOverflow=on
  Gain3 : Gain  Gain=4  Multiplication=Element-wise(K.*u)  SaturateOnIntegerOverflow=on
  Gain4 : Gain  Gain=5  Multiplication=Element-wise(K.*u)  SaturateOnIntegerOverflow=on
  Gain5 : Gain  Gain=6  Multiplication=Element-wise(K.*u)  SaturateOnIntegerOverflow=on
  ItCapTransShip : Subsystem  TreatAsAtomicUnit=on
      settings: RTWFcnNameOpts=Auto  RTWFileNameOpts=Auto
  ItJacobi : Subsystem  TreatAsAtomicUnit=on
      settings: RTWFcnNameOpts=Auto  RTWFileNameOpts=Auto
  Logical Operator2 : Logic  Operator=AND  Inputs=2
  MessageDisplay : Subsystem  TreatAsAtomicUnit=on
      settings: RTWFcnNameOpts=Auto  RTWFileNameOpts=Auto
  Mux2 : Mux  Inputs=2
  Relational Operator{,1..5} (6 alike) : RelationalOperator  Operator===
  Relational Operator6 : RelationalOperator  Operator=~=
  Relational Operator7 : RelationalOperator  Operator=~=
  Relative Bennifits : Subsystem  TreatAsAtomicUnit=on
      settings: RTWFcnNameOpts=Auto  RTWFileNameOpts=Auto
  Sum : Sum  Inputs=++++++  SaturateOnIntegerOverflow=on
  TimeLastReplan : DataStoreWrite  DataStoreName=TimeLastReplan  SampleTime=g_SampleTime
  Local Assignment : Outport  Port=1
  Algorithm Data : Outport  Port=2
  AuctionData : Outport  Port=3
  NewAssignmetTime : Outport  Port=4
  wires:
  Enable/1 -> DistAuctItCapTransShip/4(EnableType), DistItCapTransShip/4(EnableType)
  Logical Operator2/1 -> MessageDisplay/Enable
  Relational Operator7/1 -> Logical Operator2/2
  Relational Operator6/1 -> Logical Operator2/1
  Constant13/1 -> Relational Operator7/2
  Constant12/1 -> Relational Operator7/1
  Constant15/1 -> Relational Operator6/2
  Constant14/1 -> Relational Operator6/1
  DistAuctItCapTransShip/2(AuctionData) -> AuctionData/1
  Gain5/1 -> Sum/6
  DistAuctItCapTransShip/1(Local Assignment) -> Assignment  Algorithm Switch/7
  Constant11/1 -> Relational Operator5/2
  Constant10/1 -> Relational Operator5/1
  Relational Operator5/1 -> DistAuctItCapTransShip/Enable, Gain5/1
  DistItCapTransShip/2(Algorithm Data) -> Algorithm Data/1
  DistItCapTransShip/1(Local Assignment) -> Assignment  Algorithm Switch/6
  Gain4/1 -> Sum/5
  Constant9/1 -> Relational Operator4/2
  Constant8/1 -> Relational Operator4/1
  Relational Operator4/1 -> DistItCapTransShip/Enable, Gain4/1
  Bus Selector/1 -> Mux2/2  "<VehicleID>"
  Mux2/1 -> MessageDisplay/1(In1)
  SimBusIn/1 -> DistAuctItCapTransShip/3(SimBusIn), DistItCapTransShip/3(SimBusIn), Relative Bennifits/3(SimBusIn), ItJacobi/3(SimBusIn), ItCapTransShip/3(SimBusIn)
  Demux/2 -> Bus Creator1/2  "Task Assignment  - Local"
  Demux/1 -> Bus Creator1/1  "Target Assignment - Local"
  Bus Creator1/1 -> Bus Creator/1  "Assignment - Local"
  Assignment  Algorithm Switch/1 -> Demux/1
  Gain3/1 -> Sum/4
  Constant7/1 -> Relational Operator3/2
  Constant6/1 -> Relational Operator3/1
  Relational Operator3/1 -> Relative Bennifits/Enable, Gain3/1
  Relative Bennifits/1(Local Assignment) -> Assignment  Algorithm Switch/5
  Gain/1 -> Sum/3
  Gain1/1 -> Sum/2
  Gain2/1 -> Sum/1
  Sum/1 -> Assignment  Algorithm Switch/1
  Constant5/1 -> Relational Operator2/2
  Constant4/1 -> Relational Operator2/1
  Relational Operator2/1 -> ItJacobi/Enable, Gain/1
  ItJacobi/1(Local Assignment) -> Assignment  Algorithm Switch/4
  Constant3/1 -> Relational Operator1/2
  Constant2/1 -> Relational Operator1/1
  Relational Operator1/1 -> Gain1/1, ItCapTransShip/Enable
  ItCapTransShip/1(Local Assignment) -> Assignment  Algorithm Switch/3
  Constant1/1 -> Relational Operator/2
  Constant/1 -> Relational Operator/1
  Relational Operator/1 -> Gain2/1, CapTransShip/Enable
  ComBusLocalIn/1 -> Bus Selector/1, CapTransShip/1(ComBusLocalIn), DistItCapTransShip/1(ComBusLocalIn), DistAuctItCapTransShip/1(ComBusLocalIn), Relative Bennifits/1(ComBusLocalIn), ItJacobi/1(ComBusLocalIn), ItCapTransShip/1(ComBusLocalIn)
  CapTransShip/1(Local Assignment) -> Assignment  Algorithm Switch/2
  Bus Creator/1 -> Bus Creator2/2  "Assignments"
  ComBusIn/1 -> DistItCapTransShip/2(ComBusIn), DistAuctItCapTransShip/2(ComBusIn), Relative Bennifits/2(ComBusIn), ItJacobi/2(ComBusIn), ItCapTransShip/2(ComBusIn), CapTransShip/2(ComBusIn)
  Digital Clock/1 -> Mux2/1, TimeLastReplan/1, Bus Creator2/1  "CurrentTime"
  Bus Creator2/1 -> Local Assignment/1  "Assignment"
  Demux/3 -> NewAssignmetTime/1  "NewAssignmetTime"

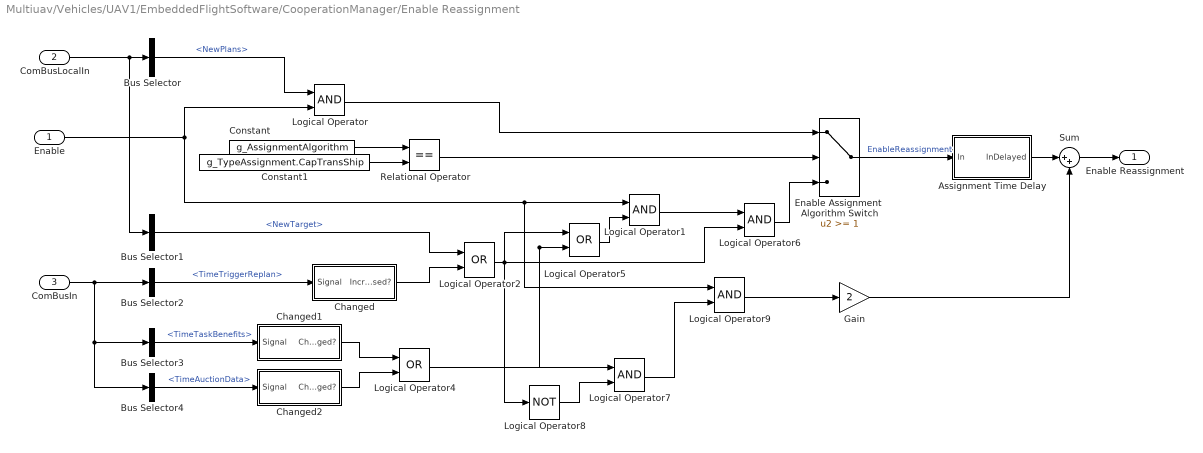
== system Multiuav/Vehicles/UAV1/EmbeddedFlightSoftware/CooperationManager/Enable Reassignment ==
  Enable : Inport  Port=1  LatchInput=off  SampleTime=g_SampleTime
  ComBusLocalIn : Inport  Port=2  LatchInput=off  SampleTime=g_SampleTime
  ComBusIn : Inport  Port=3  LatchInput=off  SampleTime=g_SampleTime
  Assignment Time Delay : Subsystem
      settings: RTWFcnNameOpts=Auto  RTWFileNameOpts=Auto
  Bus Selector : BusSelector  OutputSignals=EFS(com).RouteManager(com).NewPlans  MuxedOutput=off
  Bus Selector1 : BusSelector  OutputSignals=EFS(com).TargetManager(com).Target Status.NewTarget  MuxedOutput=off
  Bus Selector2 : BusSelector  OutputSignals=TimeTriggerReplan  MuxedOutput=off
  Bus Selector3 : BusSelector  OutputSignals=TimeTaskBenefits  MuxedOutput=off
  Bus Selector4 : BusSelector  OutputSignals=TimeAuctionData  MuxedOutput=off
  Changed : Subsystem
      settings: RTWFcnNameOpts=Auto  RTWFileNameOpts=Auto
  Changed1 : Subsystem
      settings: RTWFcnNameOpts=Auto  RTWFileNameOpts=Auto
  Changed2 : Subsystem
      settings: RTWFcnNameOpts=Auto  RTWFileNameOpts=Auto
  Constant : Constant  Value=g_AssignmentAlgorithm
  Constant1 : Constant  Value=g_TypeAssignment.CapTransShip
  Enable Assignment  Algorithm Switch : Switch  Threshold=1
  Gain : Gain  Gain=2  Multiplication=Element-wise(K.*u)  SaturateOnIntegerOverflow=on
  Logical Operator{,1,6..7,9} (5 alike) : Logic  Operator=AND  Inputs=2
  Logical Operator2 : Logic  Operator=OR  Inputs=2
  Logical Operator4 : Logic  Operator=OR  Inputs=2
  Logical Operator5 : Logic  Operator=OR  Inputs=2
  Logical Operator8 : Logic  Operator=NOT  Inputs=2
  Relational Operator : RelationalOperator  Operator===
  Sum : Sum  Inputs=|++  SaturateOnIntegerOverflow=on
  Enable Reassignment : Outport  Port=1
  wires:
  Sum/1 -> Enable Reassignment/1
  Gain/1 -> Sum/2
  Assignment Time Delay/1(InDelayed) -> Sum/1
  Logical Operator9/1 -> Gain/1
  Logical Operator7/1 -> Logical Operator9/2
  Logical Operator8/1 -> Logical Operator7/2
  Logical Operator2/1 -> Logical Operator8/1, Logical Operator6/2, Logical Operator5/1
  Logical Operator5/1 -> Logical Operator1/2
  Logical Operator4/1 -> Logical Operator5/2, Logical Operator7/1
  Changed/1(Increased?) -> Logical Operator2/2
  ComBusIn/1 -> Bus Selector2/1, Bus Selector3/1, Bus Selector4/1
  Bus Selector1/1 -> Logical Operator2/1  "<NewTarget>"
  Logical Operator/1 -> Enable Assignment  Algorithm Switch/1
  Constant1/1 -> Relational Operator/2
  Constant/1 -> Relational Operator/1
  Relational Operator/1 -> Enable Assignment  Algorithm Switch/2
  Enable/1 -> Logical Operator/2, Logical Operator1/1, Logical Operator9/1
  ComBusLocalIn/1 -> Bus Selector1/1, Bus Selector/1
  Bus Selector/1 -> Logical Operator/1  "<NewPlans>"
  Logical Operator1/1 -> Logical Operator6/1
  Bus Selector2/1 -> Changed/1(Signal)  "<TimeTriggerReplan>"
  Logical Operator6/1 -> Enable Assignment  Algorithm Switch/3
  Enable Assignment  Algorithm Switch/1 -> Assignment Time Delay/1(In)  "EnableReassignment"
  Bus Selector3/1 -> Changed1/1(Signal)  "<TimeTaskBenefits>"
  Changed1/1(Changed?) -> Logical Operator4/1
  Bus Selector4/1 -> Changed2/1(Signal)  "<TimeAuctionData>"
  Changed2/1(Changed?) -> Logical Operator4/2

== system Multiuav/Vehicles/UAV1/EmbeddedFlightSoftware/CooperationManager/Task List ==
  ComBusLocalIn : Inport  Port=1  LatchInput=off
  Bus Selector : BusSelector  OutputSignals=EFS(com).TargetManager(com).Target Status.TargetStatus  MuxedOutput=off
  Bus Selector1 : BusSelector  OutputSignals=VehicleID  MuxedOutput=off
  Check for Changed  Target Status : RelationalOperator  Operator=~=
  Constant : Constant  Value=0
  Create Last  Target Status : DataStoreMemory  DataStoreName=LastTargetStatus  InitialValue=[1:(g_MaxNumberTargets)]*-1
  Read Last  LastTargetStatus : DataStoreRead  DataStoreName=LastTargetStatus  SampleTime=g_SampleTime
  Switch : Switch  Threshold=0.5
  Update Task List : Subsystem  TreatAsAtomicUnit=on
      settings: RTWFcnNameOpts=Auto  RTWFileNameOpts=Auto
  or 1 : Logic  Operator=OR  Inputs=1
  UnassignTaskFlag : Outport  Port=1
  wires:
  Update Task List/1(UnassignedTaskFlag) -> Switch/1
  Constant/1 -> Switch/3
  Switch/1 -> UnassignTaskFlag/1
  ComBusLocalIn/1 -> Bus Selector1/1, Bus Selector/1
  Bus Selector1/1 -> Update Task List/1(Vehicle ID)  "<VehicleID>"
  or 1/1 -> Switch/2, Update Task List/Enable
  Bus Selector/1 -> Update Task List/2(TargetStatus), Check for Changed  Target Status/2  "<TargetStatus>"
  Check for Changed  Target Status/1 -> or 1/1  "ChangedTargetStatus"
  Read Last  LastTargetStatus/1 -> Check for Changed  Target Status/1  "LastTargetStatus"

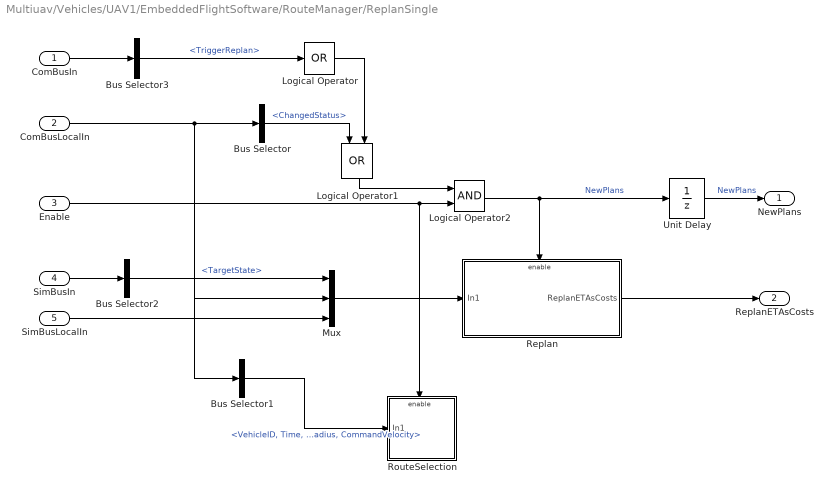
== system Multiuav/Vehicles/UAV1/EmbeddedFlightSoftware/RouteManager/ReplanSingle ==
  ComBusIn : Inport  Port=1  LatchInput=off
  ComBusLocalIn : Inport  Port=2  LatchInput=off
  Enable : Inport  Port=3  LatchInput=off
  SimBusIn : Inport  Port=4  LatchInput=off
  SimBusLocalIn : Inport  Port=5  LatchInput=off
  Bus Selector : BusSelector  OutputSignals=EFS(com).TargetManager(com).Target Status.ChangedStatus  MuxedOutput=off
  Bus Selector1 : BusSelector  OutputSignals="VehicleID,Time,EFS(com).CooperationManager(com).Assignment.Assignments.Assignment - Local.Target Assignment - Local,EFS(com).CooperationManager(com).Assignment.Assignments.Assignment - Local.Task Assignment  - Local,Dynamics(com).TacticalManuevering.WayPointNumber,EFS(com).RouteManager(com).TaskStatus.Task Finished,Dynamics(com).AC Dynamics.Position_x,Dynamics(com).AC Dynamics.Position_y,Dynamics(com).AC Dynamics.Altitude,Dynamics(com).AC Dynamics.Psi,Dynamics(com).AC Dynamics.V North,Dynamics(com).AC Dynamics.V East,Dynamics(com).TacticalManuevering.CommandTurnRadius,Dynamics(com).TacticalManuevering.CommandVelocity"  MuxedOutput=on
  Bus Selector2 : BusSelector  OutputSignals=ExternalTruth.TargetState  MuxedOutput=off
  Bus Selector3 : BusSelector  OutputSignals=TriggerReplan  MuxedOutput=off
  Logical Operator : Logic  Operator=OR  Inputs=1
  Logical Operator1 : Logic  Orientation=down  Operator=OR  Inputs=2
  Logical Operator2 : Logic  Operator=AND  Inputs=2
  Mux : Mux  Inputs=3
  Replan : Subsystem  TreatAsAtomicUnit=on
      settings: RTWFcnNameOpts=Auto  RTWFileNameOpts=Auto
  RouteSelection : Subsystem  TreatAsAtomicUnit=on
      settings: RTWFcnNameOpts=Auto  RTWFileNameOpts=Auto
  Unit Delay : UnitDelay  X0=0  SampleTime=g_SampleTime
      settings: RTWStateStorageClass=Auto
  NewPlans : Outport  Port=1
  ReplanETAsCosts : Outport  Port=2
  wires:
  Bus Selector3/1 -> Logical Operator/1  "<TriggerReplan>"
  SimBusLocalIn/1 -> Mux/3
  Replan/1(ReplanETAsCosts) -> ReplanETAsCosts/1
  SimBusIn/1 -> Bus Selector2/1
  Unit Delay/1 -> NewPlans/1  "NewPlans"
  ComBusIn/1 -> Bus Selector3/1
  ComBusLocalIn/1 -> Bus Selector1/1, Mux/2, Bus Selector/1
  Logical Operator2/1 -> Replan/Enable, Unit Delay/1  "NewPlans"
  Enable/1 -> Logical Operator2/2, RouteSelection/Enable
  Bus Selector1/1 -> RouteSelection/1(In1)  "<VehicleID, Time, Target Assignment - Local, Task Assignment  - Local, WayPointNumber, Task Finished, Position_x, Position_y, Altitude, Psi, V North, V East, CommandTurnRadius, CommandVelocity>"
  Logical Operator1/1 -> Logical Operator2/1
  Logical Operator/1 -> Logical Operator1/2
  Bus Selector/1 -> Logical Operator1/1  "<ChangedStatus>"
  Bus Selector2/1 -> Mux/1  "<TargetState>"
  Mux/1 -> Replan/1(In1)
